simulink model "regulador_y_seguidor"  (R2013a)
settings: Solver=ode45  StartTime=0.0  StopTime=5  RelTol=1e-3
settings Model: Creator=JUAN JOSE  LastModifiedBy=JUAN JOSE

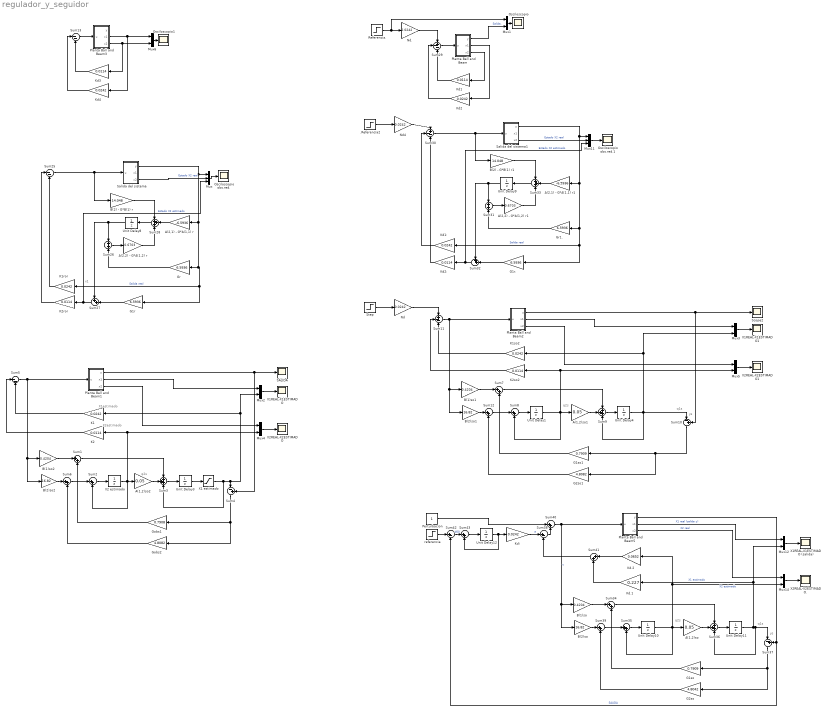
== system regulador_y_seguidor ==
  note: X1estimado
  note: X2estimado
  note: q2s
  note: q2s
  note: ys
  note: q1s
  note: x1
  note: q2s
  note: ys
  note: q1s
  .Referencia2 : Step  Time=0  After=20
  A(1,2)so : Gain  Gain=0.05
  A(1,2)so1 : Gain  Gain=0.05
  A(1,2)so2 : Gain  Gain=0.05
  A(2,1) - G*A(1,1) r : Gain  Gain=-6.5936
  A(2,1) - G*A(1,1) r1 : Gain  Gain=-6.5936
  A(2,2) - G*A(1,2) r : Gain  Gain=0.6703
  A(2,2) - G*A(1,2) r1 : Gain  Gain=0.6703
  B(1)so : Gain  Gain=0.4204
  B(1)so1 : Gain  Gain=0.4204
  B(1)so2 : Gain  Gain=0.4204
  B(2) - G*B(1) r : Gain  Gain=14.048
  B(2) - G*B(1) r1 : Gain  Gain=14.048
  B(2)so : Gain  Gain=16.82
  B(2)so1 : Gain  Gain=16.82
  B(2)so2 : Gain  Gain=16.82
  G1r : Gain  Gain=6.5936
  G1r. : Gain  Gain=6.5936
  G1so : Gain  Gain=0.7909
  G1so1 : Gain  Gain=0.7909
  G2so : Gain  Gain=4.8042
  G2so1 : Gain  Gain=4.8082
  Gobs1 : Gain  Gain=0.7908
  Gobs2 : Gain  Gain=4.8082
  Gr : Gain  Gain=6.5936
  Gr1. : Gain  Gain=6.5936
  K1 : Gain  Gain=0.0242
  K1ror : Gain  Gain=0.0242
  K1so2 : Gain  Gain=0.0242
  K2 : Gain  Gain=0.0114
  K2ror : Gain  Gain=0.0114
  K2so2 : Gain  Gain=0.0114
  Kd.1 : Gain  Gain=0.227
  Kd.2 : Gain  Gain=0.0652
  Kd1 : Gain  Gain=0.0114
  Kd1: : Gain  Gain=0.0242
  Kd2 : Gain  Gain=0.0242
  Kd2: : Gain  Gain=0.0114
  Kd3 : Gain  Gain=0.0114
  Kd4 : Gain  Gain=0.0242
  Kdi : Gain  Gain=0.0242
  Mux : Mux  Inputs=3
  Mux{1..6,12,14} (8 alike) : Mux  Inputs=2
  Mux11 : Mux  Inputs=3
  Nd : Gain  Gain=0.0242
  Nd. : Gain  Gain=0.0242
  Nd4 : Gain  Gain=0.0242
  Osciloscopio : Scope
      settings: ShowLegends=on  YMin=-30  YMax=25  SaveName=ScopeData2
  Osciloscopio obs.red. : Scope
      settings: ShowLegends=on  SaveName=ScopeData14
  Osciloscopio obs.red.1 : Scope
      settings: ShowLegends=on
  Osciloscopio1 : Scope
      settings: ShowLegends=on  YMin=-30  YMax=25  SaveName=ScopeData8
  Perturbacion : Constant
  Planta Ball and Beam : Subsystem
  Planta Ball and Beam1 : Subsystem
  Planta Ball and Beam2 : Subsystem
  Planta Ball and Beam3 : Subsystem
  Planta Ball and Beam5 : Subsystem
  Referencia. : Step  Time=0  Before=5  After=20  SampleTime=0
  SALIDA : Scope
  Salida del sistema : Subsystem
  Salida del sistema1 : Subsystem
  Scope2 : Scope
      settings: SaveName=ScopeData5
  Step : Step  Time=0  After=20  SampleTime=0
  Sum{1..2,6..8,12,34..35,39..41,43} (12 alike) : Sum  Inputs=|++
  Sum10 : Sum  Inputs=|-+
  Sum11 : Sum  Inputs=+--
  Sum13 : Sum  Inputs=|--
  Sum25 : Sum  Inputs=|--
  Sum26 : Sum  Inputs=+|+
  Sum27 : Sum  Inputs=++|
  Sum{3,9,28,33,36} (5 alike) : Sum  Inputs=+++
  Sum29 : Sum  Inputs=+--
  Sum30 : Sum  Inputs=+--
  Sum31 : Sum  Inputs=+|+
  Sum32 : Sum  Inputs=++|
  Sum37 : Sum  Inputs=|-+
  Sum38 : Sum  Inputs=|+-
  Sum4 : Sum  Inputs=|-+
  Sum42 : Sum  Inputs=|+-
  Sum5 : Sum  Inputs=|--
  Unit Delay{1,8..9,12} (4 alike) : UnitDelay  SampleTime=0.05
  Unit Delay10 : UnitDelay  InitialCondition=5  SampleTime=0.05
  Unit Delay11 : UnitDelay  InitialCondition=6  SampleTime=0.05
  Unit Delay3 : UnitDelay  InitialCondition=5  SampleTime=0.05
  Unit Delay4 : UnitDelay  InitialCondition=5  SampleTime=0.05
  X1 estimado : Saturate  UpperLimit=35  LowerLimit=5
  X1REAL-X1ESTIMADO : Scope
      settings: ShowLegends=on  SaveName=ScopeData3
  X1REAL-X1ESTIMADO (salida) : Scope
      settings: ShowLegends=on  SaveName=ScopeData15
  X1REAL-X1ESTIMADO1 : Scope
      settings: SaveName=ScopeData6
  X2 estimado : UnitDelay  InitialCondition=7  SampleTime=0.05
  X2REAL-X2ESTIMADO : Scope
      settings: ShowLegends=on  SaveName=ScopeData4
  X2REAL-X2ESTIMADO. : Scope
      settings: ShowLegends=on  SaveName=ScopeData17
  X2REAL-X2ESTIMADO1 : Scope
      settings: SaveName=ScopeData7
  "referencia " : Step  Time=0  After=20  SampleTime=0
  wires:
  Sum5/1 -> Planta Ball and Beam1/1(u), B(2)so2/1, B(1)so2/1
  B(2)so2/1 -> Sum6/1
  B(1)so2/1 -> Sum1/1
  Sum6/1 -> Sum2/1
  Sum2/1 -> X2 estimado/1
  Gobs1/1 -> Sum1/2
  Gobs2/1 -> Sum6/2
  Sum1/1 -> Sum3/1
  A(1,2)so2/1 -> Sum3/2
  Sum3/1 -> Unit Delay3/1
  Sum4/1 -> Gobs2/1, Gobs1/1
  Planta Ball and Beam/3(x2) -> Kd1/1
  Planta Ball and Beam/2(x1) -> Kd2/1
  Sum29/1 -> Planta Ball and Beam/1(u)
  K1/1 -> Sum5/2
  K2/1 -> Sum5/1
  Planta Ball and Beam1/1(y) -> Sum4/2, SALIDA/1
  Mux1/1 -> Osciloscopio/1
  Planta Ball and Beam1/2(x1) -> Mux2/1
  Mux2/1 -> X1REAL-X1ESTIMADO/1
  X2 estimado/1 -> Mux4/2, K2/1, A(1,2)so2/1, Sum2/2
  Planta Ball and Beam1/3(x2) -> Mux4/1
  Mux4/1 -> X2REAL-X2ESTIMADO/1
  Unit Delay3/1 -> X1 estimado/1
  Sum11/1 -> Planta Ball and Beam2/1(u), B(2)so1/1, B(1)so1/1
  B(2)so1/1 -> Sum12/1
  B(1)so1/1 -> Sum7/1
  Sum12/1 -> Sum8/1
  Sum8/1 -> Unit Delay1/1
  G1so1/1 -> Sum7/2
  G2so1/1 -> Sum12/2
  Sum7/1 -> Sum9/1
  A(1,2)so1/1 -> Sum9/2
  Sum9/1 -> Unit Delay4/1
  Sum10/1 -> G1so1/1, G2so1/1
  Planta Ball and Beam2/1(y) -> Scope2/1, Sum10/2
  Planta Ball and Beam2/2(x1) -> Mux3/1
  Mux3/1 -> X1REAL-X1ESTIMADO1/1
  Unit Delay1/1 -> Mux5/2, K2so2/1, A(1,2)so1/1, Sum8/2
  Planta Ball and Beam2/3(x2) -> Mux5/1
  Mux5/1 -> X2REAL-X2ESTIMADO1/1
  Unit Delay4/1 -> Sum10/1, Sum9/3, Mux3/2, K1so2/1
  K1so2/1 -> Sum11/3
  K2so2/1 -> Sum11/2
  Nd/1 -> Sum11/1
  Step/1 -> Nd/1
  X1 estimado/1 -> Sum4/1, Mux2/2, K1/1, Sum3/3
  K1ror/1 -> Sum25/2
  K2ror/1 -> Sum25/1
  Sum25/1 -> Salida del sistema/1(u), B(2) - G*B(1) r/1
  B(2) - G*B(1) r/1 -> Sum28/1
  Sum28/1 -> Unit Delay8/1
  A(2,1) - G*A(1,1) r/1 -> Sum28/2
  Unit Delay8/1 -> Sum27/1, Sum26/1
  Sum26/1 -> A(2,2) - G*A(1,2) r/1
  A(2,2) - G*A(1,2) r/1 -> Sum28/3
  Gr/1 -> Sum26/2
  Sum27/1 -> Mux/3, K2ror/1  "Estado X2 estimado"
  G1r/1 -> Sum27/2
  Mux/1 -> Osciloscopio obs.red./1
  Salida del sistema/1(y) -> Mux/1, Gr/1, G1r/1, K1ror/1, A(2,1) - G*A(1,1) r/1  "Salida real"
  Salida del sistema/3(x2) -> Mux/2  "Estado X2 real"
  Referencia./1 -> Mux1/1, Nd./1
  Kd1/1 -> Sum29/3
  Kd2/1 -> Sum29/2
  Nd./1 -> Sum29/1
  Planta Ball and Beam/1(y) -> Mux1/2  "Salida."
  Kd1:/1 -> Sum30/2
  Kd2:/1 -> Sum30/3
  Sum30/1 -> Salida del sistema1/1(u), B(2) - G*B(1) r1/1
  B(2) - G*B(1) r1/1 -> Sum33/1
  Sum33/1 -> Unit Delay9/1
  A(2,1) - G*A(1,1) r1/1 -> Sum33/2
  Unit Delay9/1 -> Sum32/1, Sum31/1
  Sum31/1 -> A(2,2) - G*A(1,2) r1/1
  A(2,2) - G*A(1,2) r1/1 -> Sum33/3
  Gr1./1 -> Sum31/2
  Sum32/1 -> Mux11/3, Kd2:/1  "Estado X2 estimado"
  G1r./1 -> Sum32/2
  Mux11/1 -> Osciloscopio obs.red.1/1
  Salida del sistema1/1(y) -> Mux11/1, Gr1./1, G1r./1, Kd1:/1, A(2,1) - G*A(1,1) r1/1  "Salida real"
  Salida del sistema1/3(x2) -> Mux11/2  "Estado X2 real"
  .Referencia2/1 -> Nd4/1
  Nd4/1 -> Sum30/1
  Sum40/1 -> B(2)so/1, B(1)so/1, Planta Ball and Beam5/1(u)  "u"
  B(2)so/1 -> Sum39/1
  B(1)so/1 -> Sum34/1
  Sum39/1 -> Sum35/1
  Sum35/1 -> Unit Delay10/1
  G1so/1 -> Sum34/2
  G2so/1 -> Sum39/2
  Sum34/1 -> Sum36/1
  A(1,2)so/1 -> Sum36/2
  Sum36/1 -> Unit Delay11/1
  Planta Ball and Beam5/1(y) -> Sum37/2, Sum42/2  "SALIDA"
  Sum38/1 -> Sum40/2
  Kd.2/1 -> Sum41/1
  Kd.1/1 -> Sum41/2
  Sum41/1 -> Sum38/2
  Kdi/1 -> Sum38/1  "e"
  "referencia "/1 -> Sum42/1
  Perturbacion/1 -> Sum40/1
  Sum37/1 -> G2so/1, G1so/1
  Sum43/1 -> Unit Delay12/1
  Unit Delay12/1 -> Sum43/2, Kdi/1
  Sum42/1 -> Sum43/1  "d00"
  Planta Ball and Beam5/2(x1) -> Mux12/1  "X1 real (salida y)"
  Mux12/1 -> X1REAL-X1ESTIMADO (salida)/1
  Unit Delay10/1 -> Kd.2/1, Mux14/2, A(1,2)so/1, Sum35/2  "X2 estimado"
  Planta Ball and Beam5/3(x2) -> Mux14/1  "X2 real"
  Mux14/1 -> X2REAL-X2ESTIMADO./1
  Unit Delay11/1 -> Sum37/1, Sum36/3, Mux12/2, Kd.1/1  "X1 estimado"
  Planta Ball and Beam3/3(x2) -> Mux6/2, Kd3/1
  Planta Ball and Beam3/2(x1) -> Mux6/1, Kd4/1
  Sum13/1 -> Planta Ball and Beam3/1(u)
  Mux6/1 -> Osciloscopio1/1
  Kd3/1 -> Sum13/2
  Kd4/1 -> Sum13/1

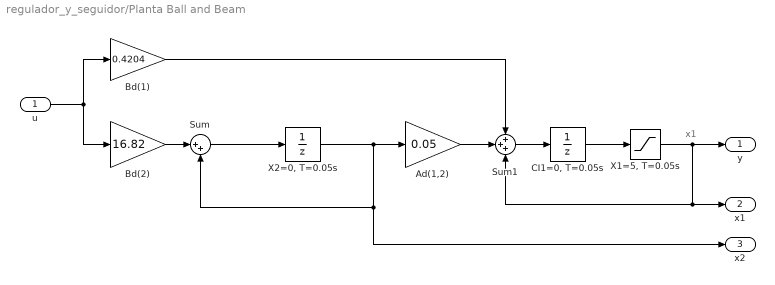
== system regulador_y_seguidor/Planta Ball and Beam ==
  note: x1
  u : Inport
  Ad(1,2) : Gain  Gain=0.05
  Bd(1) : Gain  Gain=0.4204
  Bd(2) : Gain  Gain=16.82
  "CI1=0, T=0.05s" : UnitDelay  InitialCondition=5  SampleTime=0.05
  Sum : Sum  Inputs=|++
  Sum1 : Sum  Inputs=+++
  "X1=5, T=0.05s" : Saturate  UpperLimit=35  LowerLimit=5
  "X2=0, T=0.05s" : UnitDelay  SampleTime=0.05
  y : Outport
  x1 : Outport  Port=2
  x2 : Outport  Port=3
  wires:
  u/1 -> Bd(2)/1, Bd(1)/1
  Bd(2)/1 -> Sum/1
  Ad(1,2)/1 -> Sum1/2
  Sum/1 -> "X2=0, T=0.05s"/1
  Bd(1)/1 -> Sum1/1
  Sum1/1 -> "CI1=0, T=0.05s"/1
  "CI1=0, T=0.05s"/1 -> "X1=5, T=0.05s"/1
  "X2=0, T=0.05s"/1 -> Ad(1,2)/1, x2/1, Sum/2
  "X1=5, T=0.05s"/1 -> x1/1, Sum1/3, y/1

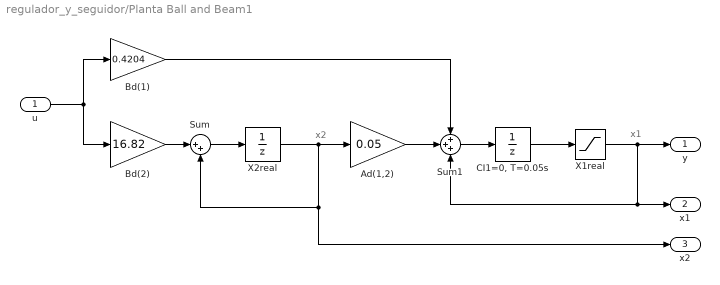
== system regulador_y_seguidor/Planta Ball and Beam1 ==
  note: x1
  note: x2
  u : Inport
  Ad(1,2) : Gain  Gain=0.05
  Bd(1) : Gain  Gain=0.4204
  Bd(2) : Gain  Gain=16.82
  "CI1=0, T=0.05s" : UnitDelay  InitialCondition=5  SampleTime=0.05
  Sum : Sum  Inputs=|++
  Sum1 : Sum  Inputs=+++
  X1real : Saturate  UpperLimit=35  LowerLimit=5
  X2real : UnitDelay  InitialCondition=10  SampleTime=0.05
  y : Outport
  x1 : Outport  Port=2
  x2 : Outport  Port=3
  wires:
  X2real/1 -> Ad(1,2)/1, x2/1, Sum/2
  u/1 -> Bd(2)/1, Bd(1)/1
  Bd(2)/1 -> Sum/1
  Ad(1,2)/1 -> Sum1/2
  Sum/1 -> X2real/1
  Bd(1)/1 -> Sum1/1
  Sum1/1 -> "CI1=0, T=0.05s"/1
  "CI1=0, T=0.05s"/1 -> X1real/1
  X1real/1 -> x1/1, Sum1/3, y/1

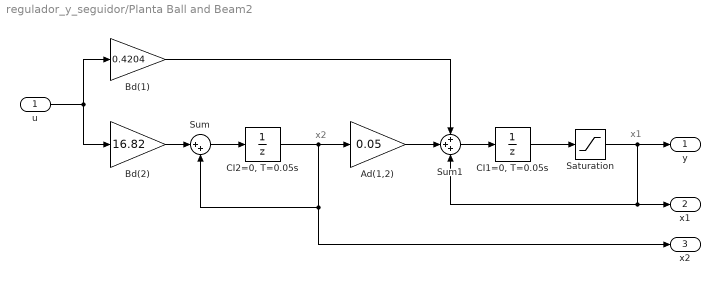
== system regulador_y_seguidor/Planta Ball and Beam2 ==
  note: x1
  note: x2
  u : Inport
  Ad(1,2) : Gain  Gain=0.05
  Bd(1) : Gain  Gain=0.4204
  Bd(2) : Gain  Gain=16.82
  "CI1=0, T=0.05s" : UnitDelay  InitialCondition=5  SampleTime=0.05
  "CI2=0, T=0.05s" : UnitDelay  SampleTime=0.05
  Saturation : Saturate  UpperLimit=35  LowerLimit=5
  Sum : Sum  Inputs=|++
  Sum1 : Sum  Inputs=+++
  y : Outport
  x1 : Outport  Port=2
  x2 : Outport  Port=3
  wires:
  "CI2=0, T=0.05s"/1 -> Ad(1,2)/1, x2/1, Sum/2
  u/1 -> Bd(2)/1, Bd(1)/1
  Bd(2)/1 -> Sum/1
  Ad(1,2)/1 -> Sum1/2
  Sum/1 -> "CI2=0, T=0.05s"/1
  Bd(1)/1 -> Sum1/1
  Sum1/1 -> "CI1=0, T=0.05s"/1
  "CI1=0, T=0.05s"/1 -> Saturation/1
  Saturation/1 -> x1/1, Sum1/3, y/1

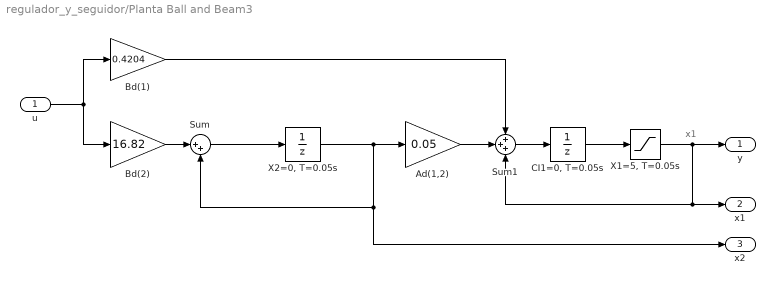
== system regulador_y_seguidor/Planta Ball and Beam3 ==
  note: x1
  u : Inport
  Ad(1,2) : Gain  Gain=0.05
  Bd(1) : Gain  Gain=0.4204
  Bd(2) : Gain  Gain=16.82
  "CI1=0, T=0.05s" : UnitDelay  InitialCondition=5  SampleTime=0.05
  Sum : Sum  Inputs=|++
  Sum1 : Sum  Inputs=+++
  "X1=5, T=0.05s" : Saturate  UpperLimit=35  LowerLimit=5
  "X2=0, T=0.05s" : UnitDelay  SampleTime=0.05
  y : Outport
  x1 : Outport  Port=2
  x2 : Outport  Port=3
  wires:
  u/1 -> Bd(2)/1, Bd(1)/1
  Bd(2)/1 -> Sum/1
  Ad(1,2)/1 -> Sum1/2
  Sum/1 -> "X2=0, T=0.05s"/1
  Bd(1)/1 -> Sum1/1
  Sum1/1 -> "CI1=0, T=0.05s"/1
  "CI1=0, T=0.05s"/1 -> "X1=5, T=0.05s"/1
  "X2=0, T=0.05s"/1 -> Ad(1,2)/1, x2/1, Sum/2
  "X1=5, T=0.05s"/1 -> x1/1, Sum1/3, y/1

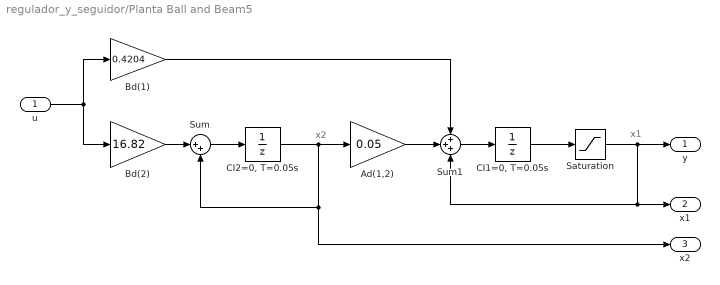
== system regulador_y_seguidor/Planta Ball and Beam5 ==
  note: x1
  note: x2
  u : Inport
  Ad(1,2) : Gain  Gain=0.05
  Bd(1) : Gain  Gain=0.4204
  Bd(2) : Gain  Gain=16.82
  "CI1=0, T=0.05s" : UnitDelay  InitialCondition=5  SampleTime=0.05
  "CI2=0, T=0.05s" : UnitDelay  SampleTime=0.05
  Saturation : Saturate  UpperLimit=35  LowerLimit=5
  Sum : Sum  Inputs=|++
  Sum1 : Sum  Inputs=+++
  y : Outport
  x1 : Outport  Port=2
  x2 : Outport  Port=3
  wires:
  "CI2=0, T=0.05s"/1 -> Ad(1,2)/1, x2/1, Sum/2
  u/1 -> Bd(2)/1, Bd(1)/1
  Bd(2)/1 -> Sum/1
  Ad(1,2)/1 -> Sum1/2
  Sum/1 -> "CI2=0, T=0.05s"/1
  Bd(1)/1 -> Sum1/1
  Sum1/1 -> "CI1=0, T=0.05s"/1
  "CI1=0, T=0.05s"/1 -> Saturation/1
  Saturation/1 -> x1/1, Sum1/3, y/1

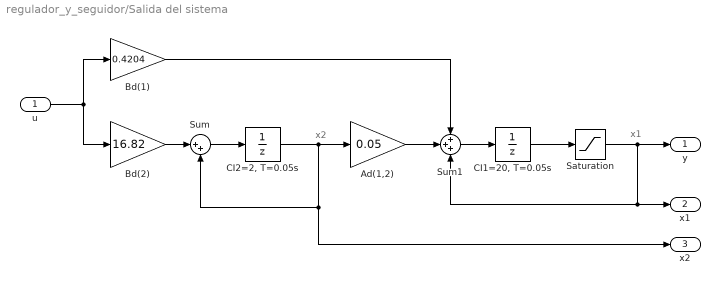
== system regulador_y_seguidor/Salida del sistema ==
  note: x1
  note: x2
  u : Inport
  Ad(1,2) : Gain  Gain=0.05
  Bd(1) : Gain  Gain=0.4204
  Bd(2) : Gain  Gain=16.82
  "CI1=20, T=0.05s" : UnitDelay  InitialCondition=20  SampleTime=0.05
  "CI2=2, T=0.05s" : UnitDelay  InitialCondition=100  SampleTime=0.05
  Saturation : Saturate  UpperLimit=35  LowerLimit=5
  Sum : Sum  Inputs=|++
  Sum1 : Sum  Inputs=+++
  y : Outport
  x1 : Outport  Port=2
  x2 : Outport  Port=3
  wires:
  "CI2=2, T=0.05s"/1 -> Ad(1,2)/1, x2/1, Sum/2
  u/1 -> Bd(2)/1, Bd(1)/1
  Bd(2)/1 -> Sum/1
  Ad(1,2)/1 -> Sum1/2
  Sum/1 -> "CI2=2, T=0.05s"/1
  Bd(1)/1 -> Sum1/1
  Sum1/1 -> "CI1=20, T=0.05s"/1
  "CI1=20, T=0.05s"/1 -> Saturation/1
  Saturation/1 -> x1/1, Sum1/3, y/1

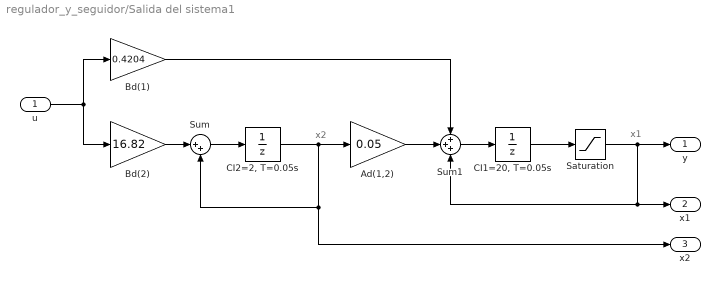
== system regulador_y_seguidor/Salida del sistema1 ==
  note: x1
  note: x2
  u : Inport
  Ad(1,2) : Gain  Gain=0.05
  Bd(1) : Gain  Gain=0.4204
  Bd(2) : Gain  Gain=16.82
  "CI1=20, T=0.05s" : UnitDelay  InitialCondition=5  SampleTime=0.05
  "CI2=2, T=0.05s" : UnitDelay  SampleTime=0.05
  Saturation : Saturate  UpperLimit=35  LowerLimit=5
  Sum : Sum  Inputs=|++
  Sum1 : Sum  Inputs=+++
  y : Outport
  x1 : Outport  Port=2
  x2 : Outport  Port=3
  wires:
  "CI2=2, T=0.05s"/1 -> Ad(1,2)/1, x2/1, Sum/2
  u/1 -> Bd(2)/1, Bd(1)/1
  Bd(2)/1 -> Sum/1
  Ad(1,2)/1 -> Sum1/2
  Sum/1 -> "CI2=2, T=0.05s"/1
  Bd(1)/1 -> Sum1/1
  Sum1/1 -> "CI1=20, T=0.05s"/1
  "CI1=20, T=0.05s"/1 -> Saturation/1
  Saturation/1 -> x1/1, Sum1/3, y/1
